simulink model "controllo_disco_rigido_rumore"  (R2019b)
settings: Solver=VariableStepAuto  StartTime=0.0  StopTime=5  FixedStep=0.01  RelTol=1e-3
values from neighbouring files (symbols this model uses):
  b = 0.002    [controllo_disco_rigido.m]    (also in controllo_disco_rigido_baseWS.mat; controllo_disco_rigido_script.m; init_controllo_disco_rigido.m)
  J = 0.001    [controllo_disco_rigido.m]    (also in controllo_disco_rigido_baseWS.mat; controllo_disco_rigido_script.m; init_controllo_disco_rigido.m)
  R1_n = 35000    [controllo_disco_rigido_script.m]
  R2_pole_n = [-500, -1400]    [controllo_disco_rigido_script.m]
  R2_zero_n = [-2]    [controllo_disco_rigido_script.m]
  y0 = 300    [controllo_disco_rigido.m]    (also in controllo_disco_rigido_script.m)
settings Model: Creator=Utente  LastModifiedBy=Utente
settings DataIOCC: SaveOutput=off  SignalLogging=off  DSMLogging=off  ReturnWorkspaceOutputsName=Mdlcl

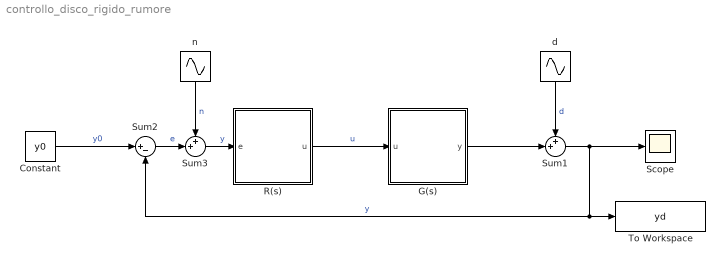
== system controllo_disco_rigido_rumore ==
  Constant : Constant  Value=y0
  G(s) : Subsystem
  R(s) : Subsystem
  Scope : Scope
  Sum1 : Sum  Inputs=++|
  Sum2 : Sum  Inputs=|+-
  Sum3 : Sum  Inputs=++|
  To Workspace : ToWorkspace  VariableName=yd  SampleTime=-1
  d : Sin  Frequency=[5]  SampleTime=0
  n : Sin  Frequency=[50]  SampleTime=0
  wires:
  R(s)/1(u) -> G(s)/1(u)  "u"
  Sum1/1 -> Scope/1, Sum2/2, To Workspace/1  "y"
  Constant/1 -> Sum2/1  "y0"
  d/1 -> Sum1/1  "d"
  G(s)/1(y) -> Sum1/2
  n/1 -> Sum3/1  "n"
  Sum2/1 -> Sum3/2  "e"
  Sum3/1 -> R(s)/1(e)  "y"

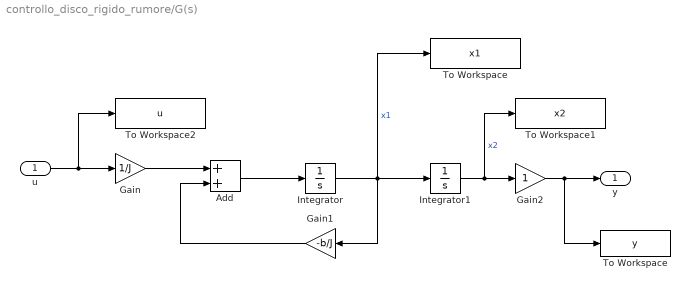
== system controllo_disco_rigido_rumore/G(s) ==
  u : Inport
  " To Workspace" : ToWorkspace  VariableName=y  SampleTime=-1
  Add : Sum
  Gain : Gain  Gain=1/J
  Gain1 : Gain  Gain=-b/J
  Gain2 : Gain
  Integrator : Integrator
  Integrator1 : Integrator
  To Workspace : ToWorkspace  VariableName=x1  SampleTime=-1
  To Workspace1 : ToWorkspace  VariableName=x2  SampleTime=-1
  To Workspace2 : ToWorkspace  VariableName=u  SampleTime=-1
  y : Outport
  wires:
  Integrator/1 -> To Workspace/1, Gain1/1, Integrator1/1  "x1"
  u/1 -> Gain/1, To Workspace2/1
  Add/1 -> Integrator/1
  Gain/1 -> Add/1
  Gain1/1 -> Add/2
  Integrator1/1 -> Gain2/1, To Workspace1/1  "x2"
  Gain2/1 -> " To Workspace"/1, y/1

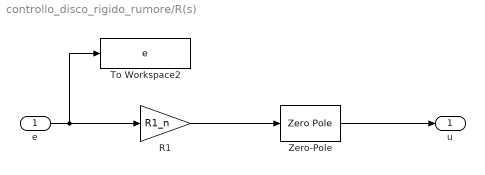
== system controllo_disco_rigido_rumore/R(s) ==
  e : Inport
  R1 : Gain  Gain=R1_n
  To Workspace2 : ToWorkspace  VariableName=e  SampleTime=-1
  Zero-Pole : ZeroPole  Zeros=R2_zero_n  Poles=R2_pole_n
  u : Outport
  wires:
  Zero-Pole/1 -> u/1
  R1/1 -> Zero-Pole/1
  e/1 -> To Workspace2/1, R1/1
